simulink model "HeatCupMain"  (R2015a)
settings: Solver=FixedStepDiscrete  StartTime=0.0  StopTime=10.0  FixedStep=dT  RelTol=1e-3
values from neighbouring files (symbols this model uses):
  dT = 0.01    [Parameters.m]
  Par_HeatCupDurationMaxTime = 7200    [Parameters.m]
  Par_TempPTCMax = 58    [Parameters.m]
  SW_OFF = SIG_HIGH    (= 1)    [Parameters.m]
  SW_ON = SIG_LOW    (= 0)    [Parameters.m]
undefined symbols (not defined in the file or in its folder): sigbuilder_block
settings Model: Creator=Daedong  LastModifiedBy=Daedong

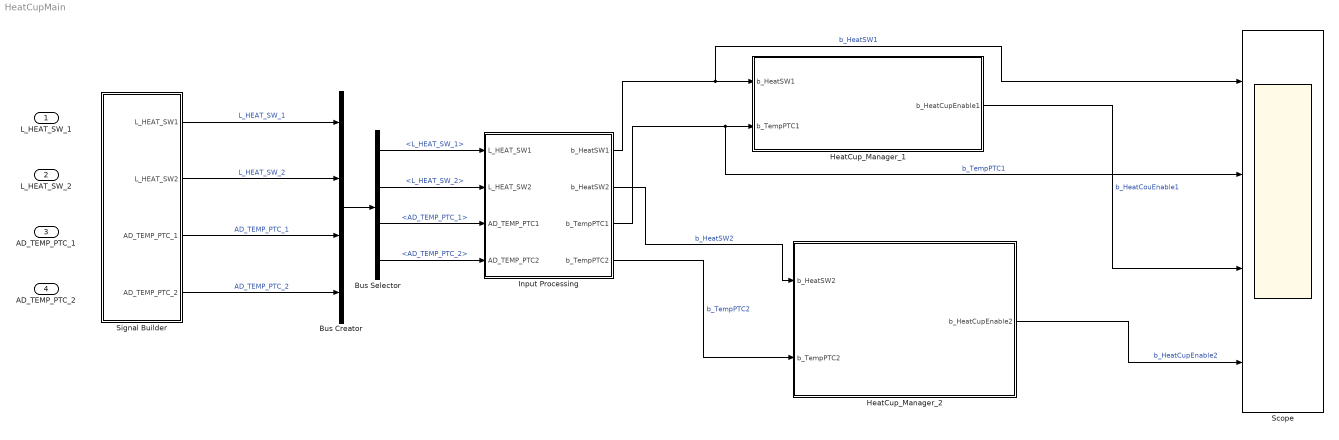
== system HeatCupMain ==
  L_HEAT_SW_1 : Inport
  L_HEAT_SW_2 : Inport  Port=2
  AD_TEMP_PTC_1 : Inport  Port=3
  AD_TEMP_PTC_2 : Inport  Port=4
  Bus Creator : BusCreator
  Bus Selector : BusSelector  OutputSignals=L_HEAT_SW_1,L_HEAT_SW_2,AD_TEMP_PTC_1,AD_TEMP_PTC_2
  HeatCup_Manager_1 : Stateflow chart  TreatAsAtomicUnit=on
  HeatCup_Manager_2 : Stateflow chart  TreatAsAtomicUnit=on
  Input Processing : Subsystem
  Scope : Scope  NumInputPorts=4
      settings: YMin=-5~-5~-5~-5  YMax=5~5~5~5
  Signal Builder : Subsystem  Tag=STV Subsys  LoadFcn=sigbuilder_block('load',[397.5 96.75 718.5 531 ]);  StartFcn=sigbuilder_block('start');  StopFcn=sigbuilder_block('stop');  ClipboardFcn=sigbuilder_block('clipboard');  mask(Sigbuilder block){}
      mask help: Simulink:masks:SigbuilderBlock_MD
      mask init:
      | if ~strcmp(get_param(bdroot(gcbh),'SimulationStatus'),'stopped') tuvar = sigbuilder_block('maskInit'); end
      settings: CopyFcn=sigbuilder_block('copy');  DeleteFcn=sigbuilder_block('delete');  ModelCloseFcn=sigbuilder_block('modelClose');  PreSaveFcn=sigbuilder_block('preSave');  PauseFcn=sigbuilder_block('pause');  ContinueFcn=sigbuilder_block('continue');  NameChangeFcn=sigbuilder_block('namechange');  OpenFcn=sigbuilder_block('open',[437.6 199.2 550.4 400 ]);  CloseFcn=sigbuilder_block('close');
      mask Display: plot(0, 0, 100, 100,[2, 2, 32, 32, 2], [68, 8, 8, 68, 68],[32, 2], [38, 38], [32, 19, 2],[53, 60, 44], [32, 17, 17, 2],[16, 16, 31, 31]);txt = getActiveGroup(gcbh);text(2, 100, txt,'verticalAlignment', 'top');
  wires:
  Signal Builder/1(L_HEAT_SW1) -> Bus Creator/1  "L_HEAT_SW_1"
  Signal Builder/2(L_HEAT_SW2) -> Bus Creator/2  "L_HEAT_SW_2"
  Signal Builder/3(AD_TEMP_PTC_1) -> Bus Creator/3  "AD_TEMP_PTC_1"
  Signal Builder/4(AD_TEMP_PTC_2) -> Bus Creator/4  "AD_TEMP_PTC_2"
  Bus Creator/1 -> Bus Selector/1
  Bus Selector/1 -> Input Processing/1(L_HEAT_SW1)  "<L_HEAT_SW_1>"
  Bus Selector/2 -> Input Processing/2(L_HEAT_SW2)  "<L_HEAT_SW_2>"
  Bus Selector/3 -> Input Processing/3(AD_TEMP_PTC1)  "<AD_TEMP_PTC_1>"
  Bus Selector/4 -> Input Processing/4(AD_TEMP_PTC2)  "<AD_TEMP_PTC_2>"
  Input Processing/1(b_HeatSW1) -> Scope/1, HeatCup_Manager_1/1(b_HeatSW1)  "b_HeatSW1"
  Input Processing/2(b_HeatSW2) -> HeatCup_Manager_2/1(b_HeatSW2)  "b_HeatSW2"
  Input Processing/3(b_TempPTC1) -> Scope/2, HeatCup_Manager_1/2(b_TempPTC1)  "b_TempPTC1"
  Input Processing/4(b_TempPTC2) -> HeatCup_Manager_2/2(b_TempPTC2)  "b_TempPTC2"
  HeatCup_Manager_1/1(b_HeatCupEnable1) -> Scope/3  "b_HeatCouEnable1"
  HeatCup_Manager_2/1(b_HeatCupEnable2) -> Scope/4  "b_HeatCupEnable2"

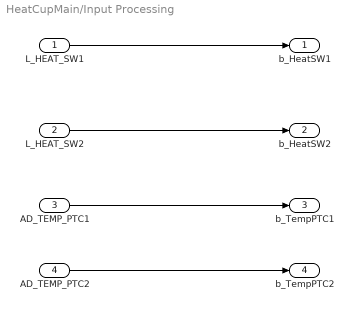
== system HeatCupMain/Input Processing ==
  L_HEAT_SW1 : Inport
  L_HEAT_SW2 : Inport  Port=2
  AD_TEMP_PTC1 : Inport  Port=3
  AD_TEMP_PTC2 : Inport  Port=4
  b_HeatSW1 : Outport
  b_HeatSW2 : Outport  Port=2
  b_TempPTC1 : Outport  Port=3
  b_TempPTC2 : Outport  Port=4
  wires:
  L_HEAT_SW1/1 -> b_HeatSW1/1
  L_HEAT_SW2/1 -> b_HeatSW2/1
  AD_TEMP_PTC1/1 -> b_TempPTC1/1
  AD_TEMP_PTC2/1 -> b_TempPTC2/1

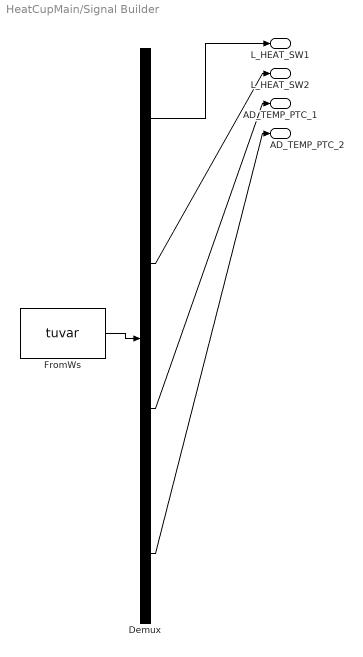
== system HeatCupMain/Signal Builder ==
  Demux : Demux  Tag=STV Demux
  FromWs : FromWorkspace  Tag=STV FromWs  VariableName=tuvar  SampleTime=0
      SigBuilderData=|
      | common.afterFinalStr = 'Extrapolate'
      | common.sampleTime = 0
      | dataSet.timeRange = [0 10]
      | dataSet.name = 'Group 1'
      | sbobj.Groups.Name = 'Group 1'
      | sbobj.Groups.Signals(1).Name = 'L_HEAT_SW1'
      | sbobj.Groups.Signals(1).XData = [0 4 4 6 6 7 7 8 8 10]
      | sbobj.Groups.Signals(1).YData = [1 1 0 0 0.98 0.98 0 0 0.98 0.98]
      | sbobj.Groups.Signals(2).Name = 'L_HEAT_SW2'
      | sbobj.Groups.Signals(2).XData = [0 10]
      | sbobj.Groups.Signals(2).YData = [0 0]
      | sbobj.Groups.Signals(3).Name = 'AD_TEMP_PTC_1'
      | sbobj.Groups.Signals(3).XData = [0 10]
      | sbobj.Groups.Signals(3).YData = [0 0]
      | sbobj.Groups.Signals(4).Name = 'AD_TEMP_PTC_2'
      | sbobj.Groups.Signals(4).XData = [0 10]
      | sbobj.Groups.Signals(4).YData = [0 0]
  L_HEAT_SW1 : Outport  Tag=STV Outport
  L_HEAT_SW2 : Outport  Tag=STV Outport  Port=2
  AD_TEMP_PTC_1 : Outport  Tag=STV Outport  Port=3
  AD_TEMP_PTC_2 : Outport  Tag=STV Outport  Port=4
  wires:
  Demux/1 -> L_HEAT_SW1/1
  FromWs/1 -> Demux/1
  Demux/2 -> L_HEAT_SW2/1
  Demux/3 -> AD_TEMP_PTC_1/1
  Demux/4 -> AD_TEMP_PTC_2/1

== stateflow chart HeatCupMain/HeatCup_Manager_2 ==
  state Main_HeatCup_Manager2 [parallel]
    settings: executionOrder=1
    state stateHeatCupOff2
    state stateHeatCupON2
    state func_STA_HeatCupOn2Off [function]
      (default) -> (junction 37) : {  b_HeatCupEnable2 = OFF;
          |    send(Cancel_Timer_HeatCupDuration2, Timer_HeatCupDuration2);  }
    (default) -> stateHeatCupOff2 : {
        | %b_HeatSW2 = SW_OFF;
        | %b_TempPTC2 = 20;
        | b_HeatCupEnable2 = OFF;
        | }
    stateHeatCupON2 -> stateHeatCupOff2 [order 1] : % 1
        | [  (b_HeatSW2 == SW_ON) && ...
        |    (b_HeatCupEnable2 == ON)  ]
        | {  func_STA_HeatCupOn2Off();  }
    stateHeatCupON2 -> stateHeatCupOff2 [order 2] : %2
        | [  (Count_HeatCupDuration2 > Par_HeatCupDurationMaxTime) ]
        | {  func_STA_HeatCupOn2Off();  }
    stateHeatCupON2 -> stateHeatCupOff2 [order 3] : %3
        | [ (b_TempPTC2 >= Par_TempPTCMax) ]
        | {  func_STA_HeatCupOn2Off();  }
    stateHeatCupOff2 -> stateHeatCupON2 : [  (b_HeatSW2 == SW_ON) && ...
        |    (b_HeatCupEnable2 == OFF) && ...
        |    (b_TempPTC2 < Par_TempPTCMax)  ]
        | {  b_HeatCupEnable2 = ON;  }
        | /  {  send(Start_Timer_HeatCupDuration2, Timer_HeatCupDuration2);  }
  state Timer_HeatCupDuration2 [parallel]
    settings: executionOrder=2
    state Timer_Off
      en:func_HeatCupDuration2_Off();
    state Timer_On
      du:func_HeatCupDuration2_On()
    state func_HeatCupDuration2_On [function]
      (default) -> (junction 17) : {Count_HeatCupDuration2=...
          |   Count_HeatCupDuration2+dT;}
    state func_HeatCupDuration2_Off [function]
      (default) -> (junction 20) : {Count_HeatCupDuration2=0;}
    (default) -> Timer_Off
    Timer_On -> Timer_Off : Cancel_Timer_HeatCupDuration2
    Timer_Off -> Timer_On : Start_Timer_HeatCupDuration2
  data: b_HeatSW2 input; b_TempPTC2 input; dT parameter; Count_HeatCupDuration2 local; Par_TempPTCMax parameter; b_HeatCupEnable2 output; Par_HeatCupDurationMaxTime parameter; SW_OFF parameter; SW_ON parameter; ON parameter; OFF parameter
  events: Start_Timer_HeatCupDuration2 local FUNCTION_CALL_EVENT; Cancel_Timer_HeatCupDuration2 local FUNCTION_CALL_EVENT

== stateflow chart HeatCupMain/HeatCup_Manager_1 ==
  state Main_HeatCup_Manager1 [parallel]
    settings: executionOrder=1
    state stateHeatCupOff1
      du:func_HeatSWDiffCheck();
    state stateHeatCupON1
      du:func_HeatSWDiffCheck();
    state func_STA_HeatCupOn2Off [function]
      (default) -> (junction 37) : {  b_HeatCupEnable1 = OFF;
          |    send(Cancel_Timer_HeatCupDuration1, Timer_HeatCupDuration1);  }
    state func_HeatSWDiffCheck [function]
      (default) -> (junction 51) : [ b_HeatSW1_Old ~= b_HeatSW1 ] {b_HeatSW1_Old = b_HeatSW1; }
    (default) -> stateHeatCupOff1 : {
        | %b_HeatSW1 = SW_OFF;
        | %b_TempPTC1 = 20;
        | b_HeatCupEnable1 = OFF;
        | b_HeatSW1_Old = SW_OFF;
        | }
    stateHeatCupON1 -> stateHeatCupOff1 [order 1] : % 1
        | [  (b_HeatSW1 == SW_ON) &&...
        |    (b_HeatCupEnable1 == ON) &&...
        |    (b_HeatSW1_Old ~= b_HeatSW1)   ]
        |  {  b_HeatSW1_Old = b_HeatSW1;
        | func_STA_HeatCupOn2Off();  }
    stateHeatCupON1 -> stateHeatCupOff1 [order 2] : %2
        | [  (Count_HeatCupDuration1 > Par_HeatCupDurationMaxTime) ]
        | /  {  func_STA_HeatCupOn2Off();  }
    stateHeatCupON1 -> stateHeatCupOff1 [order 3] : %3
        | [ (b_TempPTC1 >= Par_TempPTCMax) ]
        | /  {  func_STA_HeatCupOn2Off();  }
    stateHeatCupOff1 -> stateHeatCupON1 : %1
        | [  (b_HeatSW1 == SW_ON) &&...
        |    (b_HeatCupEnable1 == OFF) &&...
        |    (b_TempPTC1 < Par_TempPTCMax) &&...
        |    (b_HeatSW1_Old ~= b_HeatSW1)  ]
        | {  b_HeatSW1_Old = b_HeatSW1;
        | b_HeatCupEnable1 = ON;
        | send(Start_Timer_HeatCupDuration1, Timer_HeatCupDuration1);  }
  state Timer_HeatCupDuration1 [parallel]
    settings: executionOrder=2
    state Timer_Off
      en:func_HeatCupDuration1_Off();
    state Timer_On
      du:func_HeatCupDuration1_On()
    state func_HeatCupDuration1_On [function]
      (default) -> (junction 17) : {Count_HeatCupDuration1=...
          |   Count_HeatCupDuration1+dT;}
    state func_HeatCupDuration1_Off [function]
      (default) -> (junction 20) : {Count_HeatCupDuration1=0;}
    (default) -> Timer_Off
    Timer_On -> Timer_Off : Cancel_Timer_HeatCupDuration1
    Timer_Off -> Timer_On : Start_Timer_HeatCupDuration1
  data: b_HeatSW1 input; b_TempPTC1 input; dT parameter; Count_HeatCupDuration1 local; Par_TempPTCMax parameter; b_HeatCupEnable1 output; Par_HeatCupDurationMaxTime parameter; OFF parameter; SW_OFF parameter; ON parameter; SW_ON parameter; b_HeatSW1_Old local
  events: Start_Timer_HeatCupDuration1 local FUNCTION_CALL_EVENT; Cancel_Timer_HeatCupDuration1 local FUNCTION_CALL_EVENT
